simulink model "Q_4"  (R2020a)
settings: Solver=VariableStepAuto  StartTime=0.0  StopTime=10.0  RelTol=1e-3
undefined symbols (not defined in the file): b, J, k, kd, ki, kp, L, R
settings Model: DataDictionary=DC_MOTOR_DD.sldd  Creator=Admin  LastModifiedBy=Admin

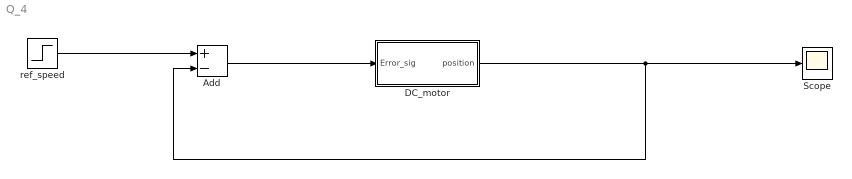
== system Q_4 ==
  Add : Sum  Inputs=+-
  DC_motor : Subsystem  TreatAsAtomicUnit=on
  Scope : Scope
  ref_speed : Step  Time=0  SampleTime=0
  wires:
  ref_speed/1 -> Add/1
  Add/1 -> DC_motor/1(Error_sig)
  DC_motor/1(position) -> Add/2, Scope/1

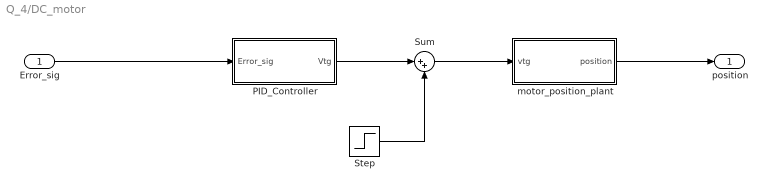
== system Q_4/DC_motor ==
  Error_sig : Inport
  PID_Controller : Subsystem  TreatAsAtomicUnit=on
  Step : Step  Time=0  Before=0.03  SampleTime=0
  Sum : Sum  Inputs=|++
  motor_position_plant : Subsystem  TreatAsAtomicUnit=on
  position : Outport
  wires:
  Step/1 -> Sum/2
  PID_Controller/1(Vtg) -> Sum/1
  Sum/1 -> motor_position_plant/1(vtg)
  Error_sig/1 -> PID_Controller/1(Error_sig)
  motor_position_plant/1(position) -> position/1

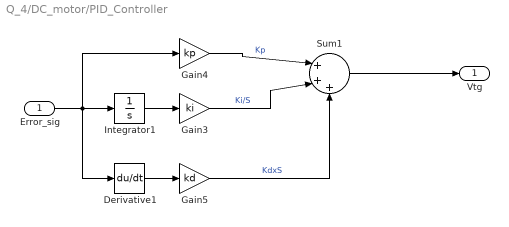
== system Q_4/DC_motor/PID_Controller ==
  Error_sig : Inport
  Derivative1 : Derivative
  Gain3 : Gain  Gain=ki
  Gain4 : Gain  Gain=kp
  Gain5 : Gain  Gain=kd
  Integrator1 : Integrator
  Sum1 : Sum  Inputs=|+++
  Vtg : Outport
  wires:
  Error_sig/1 -> Integrator1/1, Gain4/1, Derivative1/1
  Integrator1/1 -> Gain3/1
  Sum1/1 -> Vtg/1
  Derivative1/1 -> Gain5/1
  Gain3/1 -> Sum1/2  "Ki/S"
  Gain4/1 -> Sum1/1  "Kp"
  Gain5/1 -> Sum1/3  "KdxS"

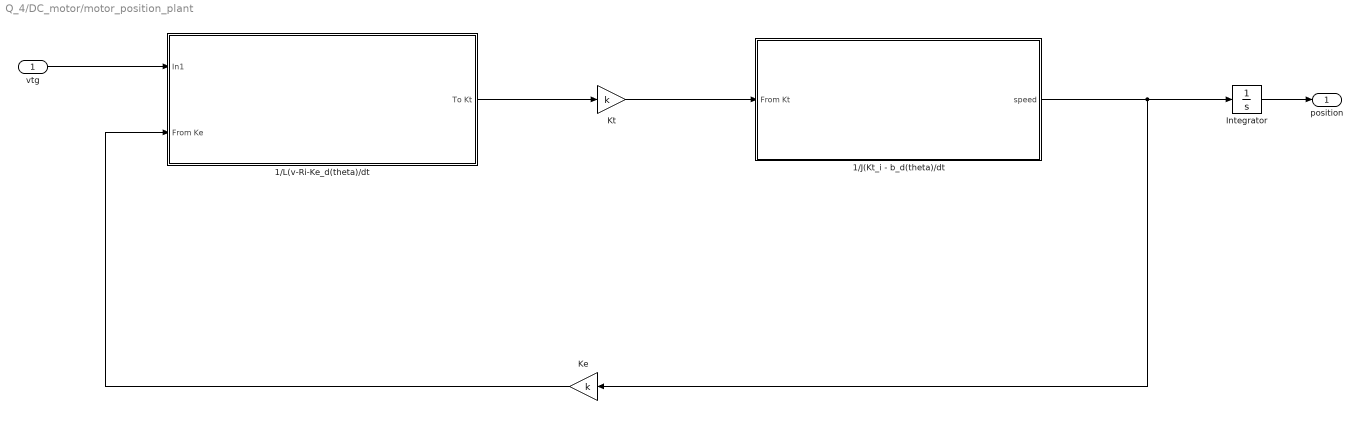
== system Q_4/DC_motor/motor_position_plant ==
  vtg : Inport
  1/J(Kt_i - b_d(theta)/dt : Subsystem
  1/L(v-Ri-Ke_d(theta)/dt : Subsystem
  Integrator : Integrator
  Ke : Gain  Gain=k
  Kt : Gain  Gain=k
  position : Outport
  wires:
  vtg/1 -> 1/L(v-Ri-Ke_d(theta)/dt/1(In1)
  Kt/1 -> 1/J(Kt_i - b_d(theta)/dt/1(From Kt)
  1/L(v-Ri-Ke_d(theta)/dt/1(To Kt) -> Kt/1
  1/J(Kt_i - b_d(theta)/dt/1(speed) -> Ke/1, Integrator/1
  Integrator/1 -> position/1
  Ke/1 -> 1/L(v-Ri-Ke_d(theta)/dt/2(From Ke)

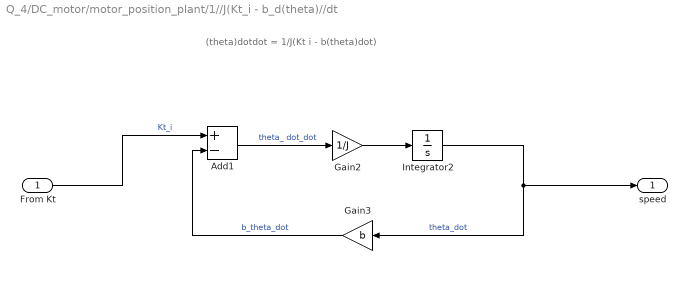
== system Q_4/DC_motor/motor_position_plant/1//J(Kt_i - b_d(theta)//dt ==
  note: (theta)dotdot = 1/J(Kt i - b(theta)dot)
  From Kt : Inport
  Add1 : Sum  Inputs=+-
  Gain2 : Gain  Gain=1/J
  Gain3 : Gain  Gain=b
  Integrator2 : Integrator
  speed : Outport
  wires:
  Gain3/1 -> Add1/2  "b_theta_dot"
  Integrator2/1 -> Gain3/1, speed/1  "theta_dot"
  Gain2/1 -> Integrator2/1
  From Kt/1 -> Add1/1  "Kt_i"
  Add1/1 -> Gain2/1  "theta_ dot_dot"

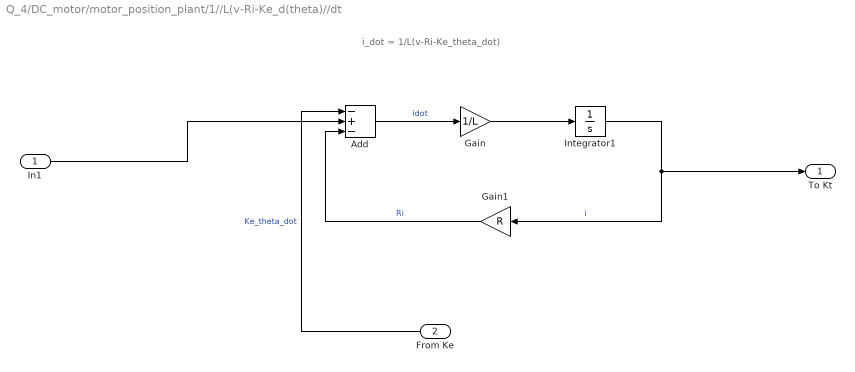
== system Q_4/DC_motor/motor_position_plant/1//L(v-Ri-Ke_d(theta)//dt ==
  note: i_dot = 1/L(v-Ri-Ke_theta_dot)
  In1 : Inport
  From Ke : Inport  Port=2
  Add : Sum  Inputs=-+-
  Gain : Gain  Gain=1/L
  Gain1 : Gain  Gain=R
  Integrator1 : Integrator
  To Kt : Outport
  wires:
  From Ke/1 -> Add/1  "Ke_theta_dot"
  In1/1 -> Add/2
  Gain1/1 -> Add/3  "Ri"
  Integrator1/1 -> Gain1/1, To Kt/1  "i"
  Add/1 -> Gain/1  "idot"
  Gain/1 -> Integrator1/1
